simulink library "ddm"  (R2021b)
settings: Solver=VariableStepAuto  StartTime=0.0  StopTime=10.0  RelTol=1e-3
undefined symbols (not defined in the file or in its folder): ENUM_ADASACCSTA_ERROR, ENUM_ADASACCSTA_OFF, ENUM_ADASACCSTA_STANDBY, ENUM_ADASISASTA_OFF, ENUM_ALLOWMOV_ALLOWREADY, ENUM_APS, ENUM_BRKSTA_ERROR, ENUM_BRKSTA_OFF, ENUM_BRKSTA_ON, ENUM_CHGPREACTERRSTA_OBCPRE, ENUM_DCDCFAULTSTA_ANYFAULTLV1, ENUM_DCDCFAULTSTA_ANYFAULTLV2, ENUM_DRIVETRAIN_AWD, ENUM_DRIVETRAIN_FWD, ENUM_DRIVETRAIN_RWD, ENUM_DRSEATSTA_INVALID, ENUM_EDUDRTSTA_NORMAL, ENUM_EPBSTA_APPLIED, ENUM_EPBSTA_RELEASED, ENUM_HVBATTREADYPRE_READY, ENUM_MCUWARN_LV0, ENUM_MCUWARN_LV1, ENUM_MCUWARN_LV2, ENUM_MCUWARN_LV3, ENUM_MCUWARN_NOERROR, ENUM_OBCFAULTSTA_ANYFAULT, ENUM_PAS_R2F2, ENUM_PDFAULT_BATTPDFAIL, ENUM_PDFAULT_DCDCDISABLE, ENUM_PDFAULT_MCUDISABLE, ENUM_PDFAULT_MCUDISCHRG, ENUM_POWERSTA_OFF, ENUM_POWERSTA_ON, ENUM_POWERSTA_READY, ENUM_POWERSTA_STANDBY, ENUM_PRESSINDI_LOW, ENUM_PUFAULT_BATTUPFAIL, ENUM_PUFAULT_DCDCENABLEFAIL, ENUM_PUFAULT_PRECHRGCHKFAIL, ENUM_PUFAULT_SAFETYCHKFAIL, ENUM_PUSTATE_COMPLETED, ENUM_PWRSTASW_OFF, ENUM_PWRSTASW_OFFA, ENUM_PWRSTASW_OFFCHVCHRG, ENUM_PWRSTASW_OFFCLVCHRG, ENUM_PWRSTASW_ON, ENUM_PWRSTASW_ONHVCHRG, ENUM_PWRSTASW_READY, ENUM_PWRSTASW_STANDBY, ENUM_RANGESTA_12IN, ENUM_RANGESTA_12OUT, ENUM_SHIFTCOMMAND_D, ENUM_SHIFTCOMMAND_N, ENUM_SHIFTCOMMAND_P, ENUM_SHIFTCOMMAND_R, ENUM_ZONEMALFUNLV_1ST, ENUM_ZONEMALFUNLV_2ND, ENUM_ZONEMALFUNLV_3RD, ENUM_ZONEMALFUNLV_4TH, ENUM_ZONESPDCTRLMODE_ACC ... (+832)
libraries: hcu_lib x738, $bdroot x26, simulink x7
(part 18 of 25)

== system ddm/DDM/DDM/PMM/SW failure/Tailgate switch failure ==
  note: Fail Safe During Detection
  note: Fail Safe After Decision
  note: Release Condition After Decision
  note: Release Condition During Detection
  note: Diagnostics and Fault Handling
  note: Test Detection Criteria
  note: Test Pass Criteria
  task_time_s : Inport
  VPMM_PowerSta_enum : Inport  Port=2
  VPMM_PwrStaSW_enum : Inport  Port=3
  VINP_TailgaSW : Inport  Port=4
  DTC_clear_request : Inport  Port=5
  Add2 : Sum
  Add3 : Sum
  Add4 : Sum  AccumDataTypeStr=uint16
  Constant{1..2,12..13,31} (5 alike) : Constant  Value=ZERO_INT
  Constant14 : Constant  Value=KDDM_TailgaSW_s
  Constant28 : Constant  Value=ZERO_FLOAT
  Constant29 : Constant  Value=ONE_INT
  Constant3 : Constant  Value=ONE_INT
  Constant37 : Constant  Value=ENUM_PWRSTASW_OFF
  Constant39 : Constant  Value=KDDM_TailgaSWPassTO_s
  Constant4 : Constant  Value=KDDM_TailgaSW_s
  Constant{42,47,52,54} (4 alike) : Constant  Value=TRUE
  Constant45 : Constant  Value=ENUM_POWERSTA_OFF
  Constant49 : Constant  Value=KDDM_TailgaSW_s
  Constant5 : Constant  Value=KDDM_TailgaSWPassTO_s
  Constant50 : Constant  Value=ENUM_PWRSTASW_OFF
  Constant53 : Constant  Value=FALSE
  Constant55 : Constant  Value=FALSE
  Constant56 : Constant  Value=KDDM_TailgaSWPassSW_flg
  Constant57 : Constant  Value=KDDM_TailgaSWCFSSW_flg
  Constant58 : Constant  Value=KDDM_TailgaSWDFSSW_flg
  Constant59 : Constant  Value=KDDM_TailgaSWDetSW_flg
  Constant6 : Constant  Value=KDDM_TailgaSWDetTO_s
  Constant60 : Constant  Value=KDDM_TailgaSWDTC_cnt
  Constant7 : Constant  Value=KDDM_TailgaSWDetTO_s
  Constant8 : Constant  Value=KDDM_TailgaSWDTC_cnt
  Constant9 : Constant  Value=FALSE
  DTC_Couter1 : hcu_lib/Basic_Blocks/DTC_Couter
  DTC_Info : hcu_lib/Basic_Blocks/DTC_Info
  Data Type Conversion : DataTypeConversion  OutDataTypeStr=uint8
  Data Type Conversion{1..2,7..9} (5 alike) : DataTypeConversion
  Data Type Conversion3 : DataTypeConversion  OutDataTypeStr=uint16
  Data Type Conversion4 : DataTypeConversion  OutDataTypeStr=uint8
  Data Type Conversion5 : DataTypeConversion  OutDataTypeStr=uint32
  Data Type Conversion6 : DataTypeConversion  OutDataTypeStr=uint16
  Divide{,1,7,11,16,20} (6 alike) : Product  Inputs=*/
  Equal10 : RelationalOperator  Operator=~=  OutDataTypeStr=boolean  RndMeth=Simplest
  Equal13 : RelationalOperator  Operator=~=  OutDataTypeStr=boolean  RndMeth=Simplest
  Equal8 : RelationalOperator  Operator===  OutDataTypeStr=boolean  RndMeth=Simplest
  Equal9 : RelationalOperator  Operator=~=  OutDataTypeStr=boolean  RndMeth=Simplest
  Logical Operator1 : Logic  Operator=NOT  AllPortsSameDT=off  OutDataTypeStr=boolean
  Logical Operator{25,28..31} (5 alike) : Logic  AllPortsSameDT=off  OutDataTypeStr=boolean
  Logical Operator27 : Logic  Operator=OR  AllPortsSameDT=off  OutDataTypeStr=boolean
  Logical Operator32 : Logic  Operator=OR  AllPortsSameDT=off  OutDataTypeStr=boolean
  Logical Operator33 : Logic  Operator=OR  AllPortsSameDT=off  OutDataTypeStr=boolean
  Relational Operator : RelationalOperator  Operator=>  OutDataTypeStr=boolean  RndMeth=Simplest
  Relational Operator1 : RelationalOperator  Operator=<=  OutDataTypeStr=boolean  RndMeth=Simplest
  Relational Operator12 : RelationalOperator  OutDataTypeStr=boolean  RndMeth=Simplest
  Relational Operator13 : RelationalOperator  Operator=<  OutDataTypeStr=boolean  RndMeth=Simplest
  Relational Operator2 : RelationalOperator  Operator=>  OutDataTypeStr=boolean  RndMeth=Simplest
  Relational Operator8 : RelationalOperator  Operator=<  OutDataTypeStr=boolean  RndMeth=Simplest
  Relational Operator9 : RelationalOperator  Operator=<=  OutDataTypeStr=boolean  RndMeth=Simplest
  Relay1 : Relay  OnSwitchValue=ONE_INT  OffSwitchValue=ZERO_INT
  SR_Latch2 : hcu_lib/Basic_Blocks/SR_Latch
  SR_Latch5 : hcu_lib/Basic_Blocks/SR_Latch
  Switch{1..3,6,8..9,13} (7 alike) : Switch  Criteria=u2 > Threshold
  Switch{4,7,11..12,15..16} (6 alike) : Switch  Criteria=u2 ~= 0
  Test Detection Criteria1 : hcu_lib/Basic_Blocks/Test Detection Criteria
  Unit Delay{1..3,5..6} (5 alike) : UnitDelay  SampleTime=-1  HasFrameUpgradeWarning=on
  VDDM_TailgaSWDTC_raw32 : Outport
  VCUTailgaSWSta : Outport  Port=2
  wires:
  DTC_clear_request/1 -> [DTC_clear_request]
  VINP_TailgaSW/1 -> [VINP_TailgaSWGPIO_flg]
  task_time_s/1 -> [task_time_s]
  [VDDM_TailgaSWCFS_flg] -> Switch11/2
  Constant42/1 -> Switch11/1
  Switch11/1 -> [VCUTailgaSWSta]
  Logical Operator27/1 -> Switch15/2
  Constant52/1 -> Switch16/1
  Equal8/1 -> Logical Operator27/1
  [VDDM_TailgaSWPass_flg] -> Switch16/2
  Constant53/1 -> Switch16/3
  Constant45/1 -> Equal8/2
  Constant55/1 -> Switch15/3
  Switch15/1 -> [VDDM_TailgaSWCFSRls_flg]
  Switch16/1 -> [VDDM_TailgaSWDFSRls_flg]
  [DTC_clear_request] -> Logical Operator27/2
  Constant54/1 -> Switch15/1
  [VPMM_PowerSta_enum] -> Equal8/1
  Relay1/1 -> SR_Latch2/1
  [VDDM_TailgaSWDet_flg] -> Logical Operator31/1
  Logical Operator29/1 -> DTC_Couter1/2
  [VDDM_TailgaSWCFSRls_flg] -> SR_Latch5/2
  SR_Latch2/1 -> Logical Operator28/2
  SR_Latch5/1 -> Logical Operator30/1
  [VDDM_TailgaSWDFSRls_flg] -> Logical Operator32/1
  Logical Operator32/1 -> SR_Latch2/2
  DTC_Couter1/2 -> Data Type Conversion4/1
  Logical Operator33/1 -> Logical Operator29/1
  Data Type Conversion4/1 -> [VDDM_TailgaSWDTC_cnt]  "VDDM_TailgaSWDTC_cnt"
  [VDDM_TailgaSWDTC_cnt] -> Relay1/1
  Logical Operator31/1 -> DTC_Couter1/1
  [VDDM_TailgaSWCFS_flg] -> Logical Operator32/2
  Constant57/1 -> Logical Operator30/2
  DTC_Couter1/1 -> SR_Latch5/1
  Constant59/1 -> Logical Operator31/2
  [VDDM_TailgaSWCFSRls_flg] -> Logical Operator33/2
  Logical Operator28/1 -> [VDDM_TailgaSWDFS_flg]
  [VDDM_TailgaSWPass_flg] -> Logical Operator33/1
  Logical Operator30/1 -> [VDDM_TailgaSWCFS_flg]
  Constant56/1 -> Logical Operator29/2
  Constant60/1 -> DTC_Couter1/3
  Constant58/1 -> Logical Operator28/1
  [VCUTailgaSWSta] -> VCUTailgaSWSta/1
  Divide1/1 -> Relational Operator1/2
  Data Type Conversion5/1 -> [VDDM_TailgaSWHiLoCount_enum]
  Relational Operator1/1 -> [VDDM_TailgaSWFailcntEN_flg]
  Divide20/1 -> Data Type Conversion9/1
  Add2/1 -> Switch6/3
  [VINP_TailgaSWGPIO_flg] -> Relational Operator/1
  Relational Operator2/1 -> Switch1/2
  Constant31/1 -> Switch6/1
  Unit Delay3/1 -> Equal10/1
  Equal10/1 -> [VDDM_TailgaSWChange_flg]
  Constant1/1 -> Switch7/3
  Constant29/1 -> Add2/2
  Switch6/1 -> Unit Delay1/1
  Unit Delay1/1 -> Data Type Conversion5/1
  Constant12/1 -> Switch1/1
  Constant37/1 -> Equal13/2
  Switch2/1 -> Data Type Conversion2/1
  Add3/1 -> Data Type Conversion8/1
  Constant4/1 -> Divide/1
  Switch9/1 -> Switch8/1
  Equal13/1 -> Switch7/2
  [VDDM_TailgaSWfail_cnt] -> Switch1/3
  [VPMM_PwrStaSW_enum] -> Equal13/1
  Switch7/1 -> Unit Delay5/1
  [VDDM_TailgaSWHiLoCount_enum] -> Relational Operator2/1
  [VDDM_TailgaSWFailcntEN_flg] -> Switch9/2
  Switch1/1 -> Switch8/3
  Test Detection Criteria1/1 -> [VDDM_TailgaSWDet_flg]  "VDDM_TailgaSWDet_flg"
  Constant7/1 -> Test Detection Criteria1/4
  [VDDM_TailgaSWHiLoCount_enum] -> Add3/1
  [VDDM_TailgaSWChange_flg] -> Switch6/2
  [VDDM_TailgaSWfail_cnt] -> Switch2/1, Relational Operator8/1
  Constant13/1 -> Switch9/3
  Constant14/1 -> Divide1/1
  Relational Operator/1 -> Unit Delay3/1, Equal10/2
  Constant28/1 -> Relational Operator/2
  Constant6/1 -> Divide20/1
  [VDDM_TailgaSWChange_flg] -> Switch8/2
  Switch8/1 -> Switch7/1
  Divide/1 -> Relational Operator2/2
  Unit Delay2/1 -> Relational Operator9/1
  Switch12/1 -> Unit Delay6/1
  Constant3/1 -> Add4/1
  Relational Operator9/1 -> Logical Operator25/2
  Data Type Conversion6/1 -> Relational Operator12/1, [VDDM_TailgaSWPass_cnt]
  [VDDM_TailgaSWChange_flg] -> Logical Operator25/1
  Switch3/1 -> Data Type Conversion3/1
  Constant2/1 -> Switch13/3
  [VDDM_TailgaSWPass_cnt] -> Switch3/1, Relational Operator13/1
  Divide11/1 -> Relational Operator12/2
  Logical Operator1/1 -> Switch13/2
  Logical Operator25/1 -> Logical Operator1/1
  Data Type Conversion/1 -> Switch12/3
  Constant5/1 -> Divide11/1
  Data Type Conversion3/1 -> Add4/2
  Add4/1 -> Switch13/1
  Equal9/1 -> Switch12/2
  Relational Operator12/1 -> [VDDM_TailgaSWPass_flg]
  Switch13/1 -> Switch12/1
  Divide7/1 -> Relational Operator9/2
  [VPMM_PwrStaSW_enum] -> Equal9/1
  Constant50/1 -> Equal9/2
  Unit Delay6/1 -> Data Type Conversion6/1
  Constant47/1 -> Data Type Conversion/1
  Constant49/1 -> Divide7/1
  Constant39/1 -> Divide16/1
  [VDDM_TailgaSWHiLoCount_enum] -> Unit Delay2/1
  VPMM_PwrStaSW_enum/1 -> [VPMM_PwrStaSW_enum]
  VPMM_PowerSta_enum/1 -> [VPMM_PowerSta_enum]
  [VINP_TailgaSWGPIO_flg] -> Switch11/3
  Data Type Conversion9/1 -> Switch2/3, Relational Operator8/2
  Relational Operator8/1 -> Switch2/2
  Data Type Conversion2/1 -> Add3/2
  [VDDM_TailgaSWHiLoCount_enum] -> Relational Operator1/1
  [VDDM_TailgaSWHiLoCount_enum] -> Add2/1
  Data Type Conversion7/1 -> [VDDM_TailgaSWfail_cnt]
  Relational Operator13/1 -> Switch3/2
  Divide16/1 -> Data Type Conversion1/1
  Data Type Conversion1/1 -> Switch3/3, Relational Operator13/2
  Data Type Conversion8/1 -> Switch9/1
  DTC_Info/1 -> VDDM_TailgaSWDTC_raw32/1  "VDDM_TailgaSWDTC_raw32"
  [VDDM_TailgaSWPass_flg] -> DTC_Info/2
  [VDDM_TailgaSWCFS_flg] -> DTC_Info/3
  [VDDM_TailgaSWDet_flg] -> DTC_Info/1
  [task_time_s] -> Divide1/2
  [task_time_s] -> Divide20/2
  [task_time_s] -> Divide/2
  [task_time_s] -> Test Detection Criteria1/2
  [task_time_s] -> Divide16/2
  [task_time_s] -> Divide7/2
  [task_time_s] -> Divide11/2
  Constant8/1 -> Test Detection Criteria1/3
  [DTC_clear_request] -> DTC_Info/4
  [DTC_clear_request] -> Switch4/2
  Switch4/1 -> Test Detection Criteria1/1
  Unit Delay5/1 -> Data Type Conversion7/1, Switch4/3
  Constant9/1 -> Switch4/1

== system ddm/DDM/DDM/PMM/System conditions of ON to READY not satisfied/SR_Latch1 ==
  set : Inport
  reset : Inport  Port=2
  Logical Operator : Logic  AllPortsSameDT=off  OutDataTypeStr=boolean
  Logical Operator1 : Logic  Operator=NOT  AllPortsSameDT=off  OutDataTypeStr=boolean
  Switch1 : Switch  Criteria=u2 ~= 0  Threshold=0.5
      settings: AttributesFormatString=<Criteria=%<Criteria>>
  Switch2 : Switch  Criteria=u2 ~= 0  Threshold=0.5
      settings: AttributesFormatString=<Criteria=%<Criteria>>
  Unit Delay : UnitDelay  SampleTime=-1  HasFrameUpgradeWarning=on
  latched : Outport
  wires:
  Logical Operator1/1 -> Switch2/1, Logical Operator/2
  Logical Operator/1 -> Switch1/2
  Switch2/1 -> Switch1/3
  Unit Delay/1 -> Switch2/3
  reset/1 -> Logical Operator1/1, Switch2/2
  set/1 -> Logical Operator/1, Switch1/1
  Switch1/1 -> latched/1, Unit Delay/1

== system ddm/DDM/DDM/PMM/power up and power down/BMS HV relay closed fail ==
  note: Release Condition After Failure Decision
  note: Test Detection Criteria
  note: Test Pass Criteria
  note: Release Condition During Failure Detection
  note: Diagnostics and Fault Handling
  note: Fail Safe Operation During Failure Detection
  note: Fail Safe Operation After Failure Decision
  task_time_s : Inport
  VPMM_PowerSta_enum : Inport  Port=2
  VPMM_PwrStaSW_enum : Inport  Port=3
  VINP_HVBContactorSta_flg : Inport  Port=4
  VPMM_PowerUpFault_enum : Inport  Port=5
  DTC_clear_request : Inport  Port=6
  VPMM_PowerUpState_enum : Inport  Port=7
  Constant : Constant  Value=ENUM_PUFAULT_BATTUPFAIL
  Constant1 : Constant  Value=ENUM_PUSTATE_COMPLETED
  Constant10 : Constant  Value=KDDM_HVRlyCloDTC_cnt
  Constant11 : Constant  Value=KDDM_HVRlyCloPassSW_flg
  Constant15 : Constant  Value=KDDM_HVRlyCloCFSSW_flg
  Constant16 : Constant  Value=TRUE
  Constant19 : Constant  Value=ENUM_POWERSTA_OFF
  Constant{2,21,25,27} (4 alike) : Constant  Value=FALSE
  Constant20 : Constant  Value=KDDM_HVRlyCloDFSSW_flg
  Constant23 : Constant  Value=TRUE
  Constant24 : Constant  Value=TRUE
  Constant26 : Constant  Value=ENUM_PWRSTASW_OFF
  Constant38 : Constant  Commented=on  Value=KDDM_HVRlyCloDetTO_s
  Constant40 : Constant  Commented=on  Value=KDDM_HVRlyCloDTC_cnt
  Constant43 : Constant  Value=KDDM_HVRlyCloPassTO_s
  Constant44 : Constant  Value=KDDM_HVRlyCloDetSW_flg
  Constant8 : Constant  Value=KDDM_HVRlyCloPassTO_s
  DTC_Couter : hcu_lib/Basic_Blocks/DTC_Couter
  DTC_Info : hcu_lib/Basic_Blocks/DTC_Info
  Data Type Conversion1 : DataTypeConversion  OutDataTypeStr=uint8
  Equal : RelationalOperator  Operator=~=  OutDataTypeStr=boolean  RndMeth=Simplest
  Equal1 : RelationalOperator  Operator===  OutDataTypeStr=boolean  RndMeth=Simplest
  Equal2 : RelationalOperator  Operator===  OutDataTypeStr=boolean  RndMeth=Simplest
  Equal5 : RelationalOperator  OutDataTypeStr=boolean  RndMeth=Simplest
  Equal6 : RelationalOperator  Operator===  OutDataTypeStr=boolean  RndMeth=Simplest
  From48 : From  Commented=on  GotoTag=task_time_s
  Goto24 : Goto  Commented=on  GotoTag=VDDM_EDriveSysErrVCUErr_flg
  Logical Operator{5,12,15,18..19} (5 alike) : Logic  AllPortsSameDT=off  OutDataTypeStr=boolean
  Logical Operator3 : Logic  Operator=OR  AllPortsSameDT=off  OutDataTypeStr=boolean
  Logical Operator4 : Logic  Operator=NOT  AllPortsSameDT=off  OutDataTypeStr=boolean
  Logical Operator6 : Logic  Operator=NOT  AllPortsSameDT=off  OutDataTypeStr=boolean
  Logical Operator8 : Logic  Operator=OR  AllPortsSameDT=off  OutDataTypeStr=boolean
  Relay : Relay  OnSwitchValue=ONE_INT  OffSwitchValue=ZERO_INT
  SR_Latch1 : Subsystem  mask(SR_Latch){}
      mask help: SR latch function.
  SR_Latch3 : hcu_lib/Basic_Blocks/SR_Latch
  SR_Latch4 : hcu_lib/Basic_Blocks/SR_Latch
  Switch{,2,4..5} (4 alike) : Switch  Criteria=u2 ~= 0
  Test Detection Criteria : hcu_lib/Basic_Blocks/Test Detection Criteria  Commented=on
  Timer1 : hcu_lib/Basic_Blocks/Timer
  VDDM_HVRlyCloDTC_raw32 : Outport
  wires:
  task_time_s/1 -> [task_time_s]
  VPMM_PwrStaSW_enum/1 -> [VPMM_PwrStaSW_enum]
  VPMM_PowerSta_enum/1 -> [VPMM_PowerSta_enum]
  Logical Operator18/1 -> [VDDM_HVRlyCloCFS_flg]
  Constant21/1 -> Switch/3
  Equal5/1 -> SR_Latch1/1(set)
  Switch4/1 -> [VDDM_HVRlyCloCFSRls_flg]
  Data Type Conversion1/1 -> [VDDM_HVRlyCloDTC_cnt]  "VDDM_HVRlyCloDTC_cnt"
  Constant8/1 -> Equal5/2
  Constant20/1 -> Logical Operator12/1
  Logical Operator12/1 -> [VDDM_HVRlyCloDFS_flg]
  Constant15/1 -> Logical Operator18/2
  [task_time_s] -> Timer1/3
  DTC_Couter/1 -> SR_Latch4/1
  [VDDM_HVRlyCloCFSRls_flg] -> Logical Operator3/2
  Logical Operator19/1 -> DTC_Couter/1
  [VPMM_PowerSta_enum] -> Equal6/1
  [VDDM_HVRlyCloPass_flg] -> Logical Operator3/1
  Constant23/1 -> Switch2/3
  Constant16/1 -> Switch/1
  Constant26/1 -> Equal/2
  SR_Latch3/1 -> Logical Operator12/2
  From48/1 -> Test Detection Criteria/2
  Switch/1 -> Goto24/1
  Switch5/1 -> [VDDM_HVRlyCloDet_flg]  "VDDM_HVRlyCloDet_flg"
  [VDDM_HVRlyCloDet_flg] -> Logical Operator19/1
  Logical Operator3/1 -> Logical Operator15/1
  Constant24/1 -> Switch4/1
  SR_Latch4/1 -> Logical Operator18/1
  Logical Operator15/1 -> DTC_Couter/2
  Constant10/1 -> DTC_Couter/3
  Constant40/1 -> Test Detection Criteria/3
  Constant25/1 -> Switch4/3
  [VPMM_PwrStaSW_enum] -> Equal/1
  Relay/1 -> SR_Latch3/1
  [VDDM_HVRlyCloCFS_flg] -> Switch/2
  [DTC_clear_request] -> Logical Operator8/2
  Constant11/1 -> Logical Operator15/2
  [VDDM_HVRlyCloDTC_cnt] -> Relay/1
  Equal2/1 -> Switch2/2
  Equal/1 -> Switch5/2
  Logical Operator8/1 -> Switch4/2
  Logical Operator6/1 -> Timer1/1
  SR_Latch1/1(latched) -> [VDDM_HVRlyCloPass_flg]
  Equal6/1 -> Logical Operator8/1
  Constant27/1 -> Switch5/3
  Constant43/1 -> Timer1/4
  DTC_Couter/2 -> Data Type Conversion1/1
  Constant44/1 -> Logical Operator19/2
  Constant19/1 -> Equal6/2
  [VDDM_HVRlyCloChk_flg] -> Switch5/1
  Timer1/1 -> Equal5/1
  Switch2/1 -> SR_Latch1/2(reset), Timer1/2, Logical Operator6/1
  [VDDM_HVRlyCloCFSRls_flg] -> SR_Latch4/2
  DTC_clear_request/1 -> [DTC_clear_request]
  Constant/1 -> Equal1/2
  Equal1/1 -> Logical Operator5/2
  Logical Operator4/1 -> Logical Operator5/1
  VINP_HVBContactorSta_flg/1 -> Logical Operator4/1
  VPMM_PowerUpFault_enum/1 -> Equal1/1
  Logical Operator5/1 -> [VDDM_HVRlyCloChk_flg]
  DTC_Info/1 -> VDDM_HVRlyCloDTC_raw32/1  "VDDM_HVRlyCloDTC_raw32"
  [VDDM_HVRlyCloPass_flg] -> DTC_Info/2
  [VDDM_HVRlyCloCFS_flg] -> DTC_Info/3
  [VDDM_HVRlyCloCFS_flg] -> SR_Latch3/2
  [VDDM_HVRlyCloDet_flg] -> DTC_Info/1
  Constant38/1 -> Test Detection Criteria/4
  [DTC_clear_request] -> DTC_Info/4
  VPMM_PowerUpState_enum/1 -> [VPMM_PowerUpState_enum]
  Constant2/1 -> Switch2/1
  Constant1/1 -> Equal2/2
  [VPMM_PowerUpState_enum] -> Equal2/1

== system ddm/DDM/DDM/PMM/power up and power down/BMS HV relay opened fail ==
  note: Test Pass Criteria
  note: Diagnostics and Fault Handling
  note: Test Detection Criteria
  note: Fail Safe Operation After Failure Decision
  note: Release Condition During Failure Detection
  note: Fail Safe Operation During Failure Detection
  note: Release Condition After Failure Decision
  task_time_s : Inport
  VPMM_PowerSta_enum : Inport  Port=2
  VPMM_PwrStaSW_enum : Inport  Port=3
  VPMM_PowerDownFault_enum : Inport  Port=4
  DTC_clear_request : Inport  Port=5
  Constant : Constant  Value=ENUM_PDFAULT_BATTPDFAIL
  Constant1 : Constant  Value=ENUM_PWRSTASW_OFF
  Constant10 : Constant  Value=KDDM_HVRlyOpDTC_cnt
  Constant11 : Constant  Value=KDDM_HVRlyOpPassSW_flg
  Constant15 : Constant  Value=KDDM_HVRlyOpCFSSW_flg
  Constant16 : Constant  Value=TRUE
  Constant17 : Constant  Value=KDDM_HVRlyOpPassTO_s
  Constant19 : Constant  Value=ENUM_POWERSTA_OFF
  Constant20 : Constant  Value=KDDM_HVRlyOpDFSSW_flg
  Constant21 : Constant  Value=FALSE
  Constant22 : Constant  Value=ENUM_PWRSTASW_OFF
  Constant23 : Constant  Value=TRUE
  Constant24 : Constant  Value=TRUE
  Constant25 : Constant  Value=FALSE
  Constant27 : Constant  Value=FALSE
  Constant38 : Constant  Commented=on  Value=KDDM_HVRlyOpDetTO_s
  Constant40 : Constant  Commented=on  Value=KDDM_HVRlyOpDTC_cnt
  Constant43 : Constant  Value=KDDM_HVRlyOpPassTO_s
  Constant44 : Constant  Value=KDDM_HVRlyOpDetSW_flg
  DTC_Couter : hcu_lib/Basic_Blocks/DTC_Couter
  DTC_Info : hcu_lib/Basic_Blocks/DTC_Info
  Data Type Conversion1 : DataTypeConversion  OutDataTypeStr=uint8
  Equal1 : RelationalOperator  Operator===  OutDataTypeStr=boolean  RndMeth=Simplest
  Equal2 : RelationalOperator  Operator=~=  OutDataTypeStr=boolean  RndMeth=Simplest
  Equal4 : RelationalOperator  Operator=~=  OutDataTypeStr=boolean  RndMeth=Simplest
  Equal6 : RelationalOperator  OutDataTypeStr=boolean  RndMeth=Simplest
  Equal7 : RelationalOperator  Operator===  OutDataTypeStr=boolean  RndMeth=Simplest
  From48 : From  Commented=on  GotoTag=task_time_s
  Logical Operator{12,15,18..19} (4 alike) : Logic  AllPortsSameDT=off  OutDataTypeStr=boolean
  Logical Operator3 : Logic  Operator=OR  AllPortsSameDT=off  OutDataTypeStr=boolean
  Logical Operator6 : Logic  Operator=NOT  AllPortsSameDT=off  OutDataTypeStr=boolean
  Logical Operator8 : Logic  Operator=OR  AllPortsSameDT=off  OutDataTypeStr=boolean
  Relay : Relay  OnSwitchValue=ONE_INT  OffSwitchValue=ZERO_INT
  SR_Latch1 : Subsystem  mask(SR_Latch){}
      mask help: SR latch function.
  SR_Latch3 : hcu_lib/Basic_Blocks/SR_Latch
  SR_Latch4 : hcu_lib/Basic_Blocks/SR_Latch
  Switch{,1,4..5} (4 alike) : Switch  Criteria=u2 ~= 0
  Test Detection Criteria : hcu_lib/Basic_Blocks/Test Detection Criteria  Commented=on
  Timer1 : hcu_lib/Basic_Blocks/Timer
  VDDM_HVRlyOpDTC_raw32 : Outport
  VDDM_HVRlyOpFail_flg : Outport  Port=2
  wires:
  task_time_s/1 -> [task_time_s]
  VPMM_PwrStaSW_enum/1 -> [VPMM_PwrStaSW_enum]
  VPMM_PowerSta_enum/1 -> [VPMM_PowerSta_enum]
  Equal4/1 -> Switch5/2
  SR_Latch1/1(latched) -> [VDDM_HVRlyOpPass_flg]
  Constant44/1 -> Logical Operator19/2
  [VDDM_HVRlyOpDTC_cnt] -> Relay/1
  Equal2/1 -> Switch1/2
  [VDDM_HVRlyOpCFSRls_flg] -> SR_Latch4/2
  DTC_Couter/2 -> Data Type Conversion1/1
  Constant20/1 -> Logical Operator12/1
  SR_Latch4/1 -> Logical Operator18/1
  Constant23/1 -> Switch1/3
  Constant11/1 -> Logical Operator15/2
  Constant17/1 -> Equal6/2
  Logical Operator15/1 -> DTC_Couter/2
  DTC_Couter/1 -> SR_Latch4/1
  Constant27/1 -> Switch5/3
  [VPMM_PwrStaSW_enum] -> Equal4/1
  [VPMM_PowerSta_enum] -> Equal7/1
  Switch4/1 -> [VDDM_HVRlyOpCFSRls_flg]
  [VDDM_HVRlyOpChk_flg] -> Switch1/1
  [VDDM_HVRlyOpCFS_flg] -> Switch/2
  Constant19/1 -> Equal7/2
  Constant21/1 -> Switch/3
  [VDDM_HVRlyOpDet_flg] -> Logical Operator19/1
  Logical Operator3/1 -> Logical Operator15/1
  [VDDM_HVRlyOpChk_flg] -> Switch5/1
  [task_time_s] -> Timer1/3
  Constant43/1 -> Timer1/4
  Constant22/1 -> Equal4/2
  Constant25/1 -> Switch4/3
  Relay/1 -> SR_Latch3/1
  Timer1/1 -> Equal6/1
  Constant10/1 -> DTC_Couter/3
  Switch1/1 -> Logical Operator6/1, SR_Latch1/2(reset), Timer1/2
  Equal6/1 -> SR_Latch1/1(set)
  Logical Operator18/1 -> [VDDM_HVRlyOpCFS_flg]
  Data Type Conversion1/1 -> [VDDM_HVRlyOpDTC_cnt]  "VDDM_HVRlyOpDTC_cnt"
  Constant24/1 -> Switch4/1
  From48/1 -> Test Detection Criteria/2
  Switch/1 -> [VDDM_HVRlyOpFail_flg]  "VDDM_HVRlyOpFail_flg"
  SR_Latch3/1 -> Logical Operator12/2
  [VDDM_HVRlyOpCFSRls_flg] -> Logical Operator3/2
  Logical Operator6/1 -> Timer1/1
  [VDDM_HVRlyOpPass_flg] -> Logical Operator3/1
  Logical Operator8/1 -> Switch4/2
  Constant40/1 -> Test Detection Criteria/3
  Switch5/1 -> [VDDM_HVRlyOpDet_flg]  "VDDM_HVRlyOpDet_flg"
  Constant1/1 -> Equal2/2
  Logical Operator12/1 -> [VDDM_HVRlyOpDFS_flg]
  Equal7/1 -> Logical Operator8/1
  [VPMM_PwrStaSW_enum] -> Equal2/1
  Constant16/1 -> Switch/1
  Constant15/1 -> Logical Operator18/2
  [DTC_clear_request] -> Logical Operator8/2
  Logical Operator19/1 -> DTC_Couter/1
  DTC_clear_request/1 -> [DTC_clear_request]
  VPMM_PowerDownFault_enum/1 -> Equal1/1
  Constant/1 -> Equal1/2
  Equal1/1 -> [VDDM_HVRlyOpChk_flg]
  [VDDM_HVRlyOpFail_flg] -> VDDM_HVRlyOpFail_flg/1
  DTC_Info/1 -> VDDM_HVRlyOpDTC_raw32/1  "VDDM_HVRlyOpDTC_raw32"
  [VDDM_HVRlyOpPass_flg] -> DTC_Info/2
  [VDDM_HVRlyOpCFS_flg] -> DTC_Info/3
  [VDDM_HVRlyOpCFS_flg] -> SR_Latch3/2
  [VDDM_HVRlyOpDet_flg] -> DTC_Info/1
  Constant38/1 -> Test Detection Criteria/4
  [DTC_clear_request] -> DTC_Info/4

== system ddm/DDM/DDM/PMM/power up and power down/BMS ready fail ==
  note: Fail Safe Operation After Failure Decision
  note: Fail Safe Operation During Failure Detection
  note: Diagnostics and Fault Handling
  note: Release Condition During Failure Detection
  note: Test Pass Criteria
  note: Test Detection Criteria
  note: Release Condition After Failure Decision
  task_time_s : Inport
  VPMM_PowerSta_enum : Inport  Port=2
  VPMM_PwrStaSW_enum : Inport  Port=3
  VINP_BMSREADY_flg : Inport  Port=4
  VPMM_PowerUpFault_enum : Inport  Port=5
  DTC_clear_request : Inport  Port=6
  VPMM_PowerUpState_enum : Inport  Port=7
  Constant : Constant  Value=ENUM_PUFAULT_BATTUPFAIL
  Constant1 : Constant  Value=ENUM_PWRSTASW_OFF
  Constant10 : Constant  Value=KDDM_BMSRdyDTC_cnt
  Constant11 : Constant  Value=KDDM_BMSRdyPassSW_flg
  Constant15 : Constant  Value=KDDM_BMSRdyCFSSW_flg
  Constant16 : Constant  Value=TRUE
  Constant19 : Constant  Value=ENUM_POWERSTA_OFF
  Constant2 : Constant  Value=ENUM_PUSTATE_COMPLETED
  Constant20 : Constant  Value=KDDM_BMSRdyDFSSW_flg
  Constant{3,21,25,27} (4 alike) : Constant  Value=FALSE
  Constant23 : Constant  Value=TRUE
  Constant24 : Constant  Value=TRUE
  Constant38 : Constant  Commented=on  Value=KDDM_BMSRdyDetTO_s
  Constant40 : Constant  Commented=on  Value=KDDM_BMSRdyDTC_cnt
  Constant43 : Constant  Value=KDDM_BMSRdyPassTO_s
  Constant44 : Constant  Value=KDDM_BMSRdyDetSW_flg
  Constant8 : Constant  Value=KDDM_BMSRdyPassTO_s
  DTC_Couter : hcu_lib/Basic_Blocks/DTC_Couter
  DTC_Info : hcu_lib/Basic_Blocks/DTC_Info
  Data Type Conversion1 : DataTypeConversion  OutDataTypeStr=uint8
  Equal : RelationalOperator  Operator=~=  OutDataTypeStr=boolean  RndMeth=Simplest
  Equal1 : RelationalOperator  Operator===  OutDataTypeStr=boolean  RndMeth=Simplest
  Equal2 : RelationalOperator  Operator===  OutDataTypeStr=boolean  RndMeth=Simplest
  Equal5 : RelationalOperator  OutDataTypeStr=boolean  RndMeth=Simplest
  Equal6 : RelationalOperator  Operator===  OutDataTypeStr=boolean  RndMeth=Simplest
  From48 : From  Commented=on  GotoTag=task_time_s
  Goto24 : Goto  Commented=on  GotoTag=VDDM_EDriveSysErrVCUErr_flg
  Logical Operator{5,12,15,18..19} (5 alike) : Logic  AllPortsSameDT=off  OutDataTypeStr=boolean
  Logical Operator3 : Logic  Operator=OR  AllPortsSameDT=off  OutDataTypeStr=boolean
  Logical Operator4 : Logic  Operator=NOT  AllPortsSameDT=off  OutDataTypeStr=boolean
  Logical Operator6 : Logic  Operator=NOT  AllPortsSameDT=off  OutDataTypeStr=boolean
  Logical Operator8 : Logic  Operator=OR  AllPortsSameDT=off  OutDataTypeStr=boolean
  Relay : Relay  OnSwitchValue=ONE_INT  OffSwitchValue=ZERO_INT
  SR_Latch1 : Subsystem  mask(SR_Latch){}
      mask help: SR latch function.
  SR_Latch3 : hcu_lib/Basic_Blocks/SR_Latch
  SR_Latch4 : hcu_lib/Basic_Blocks/SR_Latch
  Switch{,2,4..5} (4 alike) : Switch  Criteria=u2 ~= 0
  Test Detection Criteria : hcu_lib/Basic_Blocks/Test Detection Criteria  Commented=on
  Timer1 : hcu_lib/Basic_Blocks/Timer
  VDDM_BMSRdyDTC_raw32 : Outport
  wires:
  Logical Operator5/1 -> [VDDM_BMSRdyChk_flg]
  VPMM_PowerUpFault_enum/1 -> Equal1/1
  VINP_BMSREADY_flg/1 -> Logical Operator4/1
  Logical Operator4/1 -> Logical Operator5/1
  Equal1/1 -> Logical Operator5/2
  Constant/1 -> Equal1/2
  DTC_clear_request/1 -> [DTC_clear_request]
  [VDDM_BMSRdyCFSRls_flg] -> SR_Latch4/2
  Switch2/1 -> Logical Operator6/1, Timer1/2, SR_Latch1/2(reset)
  Timer1/1 -> Equal5/1
  [VDDM_BMSRdyChk_flg] -> Switch5/1
  Constant19/1 -> Equal6/2
  Constant44/1 -> Logical Operator19/2
  DTC_Couter/2 -> Data Type Conversion1/1
  Constant43/1 -> Timer1/4
  Constant27/1 -> Switch5/3
  Equal6/1 -> Logical Operator8/1
  SR_Latch1/1(latched) -> [VDDM_BMSRdyPass_flg]
  Logical Operator6/1 -> Timer1/1
  Logical Operator8/1 -> Switch4/2
  Equal/1 -> Switch5/2
  Equal2/1 -> Switch2/2
  [VDDM_BMSRdyDTC_cnt] -> Relay/1
  Constant11/1 -> Logical Operator15/2
  [DTC_clear_request] -> Logical Operator8/2
  [VDDM_BMSRdyCFS_flg] -> Switch/2
  Relay/1 -> SR_Latch3/1
  [VPMM_PwrStaSW_enum] -> Equal/1
  Constant25/1 -> Switch4/3
  Constant40/1 -> Test Detection Criteria/3
  Constant10/1 -> DTC_Couter/3
  Logical Operator15/1 -> DTC_Couter/2
  SR_Latch4/1 -> Logical Operator18/1
  Constant24/1 -> Switch4/1
  Logical Operator3/1 -> Logical Operator15/1
  [VDDM_BMSRdyDet_flg] -> Logical Operator19/1
  Switch5/1 -> [VDDM_BMSRdyDet_flg]  "VDDM_BMSRdyDet_flg"
  Switch/1 -> Goto24/1
  From48/1 -> Test Detection Criteria/2
  SR_Latch3/1 -> Logical Operator12/2
  Constant1/1 -> Equal/2
  Constant16/1 -> Switch/1
  Constant23/1 -> Switch2/3
  [VDDM_BMSRdyPass_flg] -> Logical Operator3/1
  [VPMM_PowerSta_enum] -> Equal6/1
  Logical Operator19/1 -> DTC_Couter/1
  [VDDM_BMSRdyCFSRls_flg] -> Logical Operator3/2
  DTC_Couter/1 -> SR_Latch4/1
  [task_time_s] -> Timer1/3
  Constant15/1 -> Logical Operator18/2
  Logical Operator12/1 -> [VDDM_BMSRdyDFS_flg]
  Constant20/1 -> Logical Operator12/1
  Constant8/1 -> Equal5/2
  Data Type Conversion1/1 -> [VDDM_BMSRdyDTC_cnt]  "VDDM_BMSRdyDTC_cnt"
  Switch4/1 -> [VDDM_BMSRdyCFSRls_flg]
  Equal5/1 -> SR_Latch1/1(set)
  Constant21/1 -> Switch/3
  Logical Operator18/1 -> [VDDM_BMSRdyCFS_flg]
  VPMM_PowerSta_enum/1 -> [VPMM_PowerSta_enum]
  VPMM_PwrStaSW_enum/1 -> [VPMM_PwrStaSW_enum]
  task_time_s/1 -> [task_time_s]
  DTC_Info/1 -> VDDM_BMSRdyDTC_raw32/1  "VDDM_BMSRdyDTC_raw32"
  [VDDM_BMSRdyCFS_flg] -> DTC_Info/3
  [VDDM_BMSRdyCFS_flg] -> SR_Latch3/2
  [VDDM_BMSRdyDet_flg] -> DTC_Info/1
  [VDDM_BMSRdyPass_flg] -> DTC_Info/2
  Constant38/1 -> Test Detection Criteria/4
  [DTC_clear_request] -> DTC_Info/4
  VPMM_PowerUpState_enum/1 -> [VPMM_PowerUpState_enum]
  Constant3/1 -> Switch2/1
  Constant2/1 -> Equal2/2
  [VPMM_PowerUpState_enum] -> Equal2/1

== system ddm/DDM/DDM/PMM/power up and power down/DCDC disable fail ==
  note: Fail Safe Operation After Failure Decision
  note: Fail Safe Operation During Failure Detection
  note: Diagnostics and Fault Handling
  note: Release Condition After Failure Decision
  note: Release Condition During Failure Detection
  note: Test Detection Criteria
  note: Test Pass Criteria
  task_time_s : Inport
  VPMM_PowerSta_enum : Inport  Port=2
  VPMM_PwrStaSW_enum : Inport  Port=3
  VPMM_PowerDownFault_enum : Inport  Port=4
  DTC_clear_request : Inport  Port=5
  Constant : Constant  Value=ENUM_PDFAULT_DCDCDISABLE
  Constant1 : Constant  Value=ENUM_PWRSTASW_OFF
  Constant10 : Constant  Value=KDDM_DCDCDisDTC_cnt
  Constant11 : Constant  Value=KDDM_DCDCDisPassSW_flg
  Constant15 : Constant  Value=KDDM_DCDCDisCFSSW_flg
  Constant16 : Constant  Value=TRUE
  Constant17 : Constant  Value=KDDM_DCDCDisPassTO_s
  Constant19 : Constant  Value=ENUM_POWERSTA_OFF
  Constant20 : Constant  Value=KDDM_DCDCDisDFSSW_flg
  Constant21 : Constant  Value=FALSE
  Constant22 : Constant  Value=ENUM_PWRSTASW_OFF
  Constant23 : Constant  Value=TRUE
  Constant24 : Constant  Value=TRUE
  Constant25 : Constant  Value=FALSE
  Constant27 : Constant  Value=FALSE
  Constant38 : Constant  Commented=on  Value=KDDM_DCDCDisDetTO_s
  Constant40 : Constant  Commented=on  Value=KDDM_DCDCDisDTC_cnt
  Constant43 : Constant  Value=KDDM_DCDCDisPassTO_s
  Constant44 : Constant  Value=KDDM_DCDCDisDetSW_flg
  DTC_Couter : hcu_lib/Basic_Blocks/DTC_Couter
  DTC_Info : hcu_lib/Basic_Blocks/DTC_Info
  Data Type Conversion1 : DataTypeConversion  OutDataTypeStr=uint8
  Equal1 : RelationalOperator  Operator===  OutDataTypeStr=boolean  RndMeth=Simplest
  Equal2 : RelationalOperator  Operator=~=  OutDataTypeStr=boolean  RndMeth=Simplest
  Equal4 : RelationalOperator  Operator=~=  OutDataTypeStr=boolean  RndMeth=Simplest
  Equal6 : RelationalOperator  OutDataTypeStr=boolean  RndMeth=Simplest
  Equal7 : RelationalOperator  Operator===  OutDataTypeStr=boolean  RndMeth=Simplest
  From48 : From  Commented=on  GotoTag=task_time_s
  Goto24 : Goto  Commented=on  GotoTag=VDDM_EDriveSysErrVCUErr_flg
  Logical Operator{12,15,18..19} (4 alike) : Logic  AllPortsSameDT=off  OutDataTypeStr=boolean
  Logical Operator3 : Logic  Operator=OR  AllPortsSameDT=off  OutDataTypeStr=boolean
  Logical Operator6 : Logic  Operator=NOT  AllPortsSameDT=off  OutDataTypeStr=boolean
  Logical Operator8 : Logic  Operator=OR  AllPortsSameDT=off  OutDataTypeStr=boolean
  Relay : Relay  OnSwitchValue=ONE_INT  OffSwitchValue=ZERO_INT
  SR_Latch1 : Subsystem  mask(SR_Latch){}
      mask help: SR latch function.
  SR_Latch3 : hcu_lib/Basic_Blocks/SR_Latch
  SR_Latch4 : hcu_lib/Basic_Blocks/SR_Latch
  Switch{,1,4..5} (4 alike) : Switch  Criteria=u2 ~= 0
  Test Detection Criteria : hcu_lib/Basic_Blocks/Test Detection Criteria  Commented=on
  Timer1 : hcu_lib/Basic_Blocks/Timer
  VDDM_DCDCDisDTC_raw32 : Outport
  wires:
  VPMM_PowerSta_enum/1 -> [VPMM_PowerSta_enum]
  VPMM_PwrStaSW_enum/1 -> [VPMM_PwrStaSW_enum]
  task_time_s/1 -> [task_time_s]
  Switch5/1 -> [VDDM_DCDCDisDet_flg]  "VDDM_DCDCDisDet_flg"
  Logical Operator6/1 -> Timer1/1
  Logical Operator8/1 -> Switch4/2
  [VDDM_DCDCDisCFSRls_flg] -> Logical Operator3/2
  SR_Latch3/1 -> Logical Operator12/2
  Switch/1 -> Goto24/1
  From48/1 -> Test Detection Criteria/2
  Constant24/1 -> Switch4/1
  Logical Operator18/1 -> [VDDM_DCDCDisCFS_flg]
  Constant15/1 -> Logical Operator18/2
  Constant21/1 -> Switch/3
  [VDDM_DCDCDisDet_flg] -> Logical Operator19/1
  Data Type Conversion1/1 -> [VDDM_DCDCDisDTC_cnt]  "VDDM_DCDCDisDTC_cnt"
  Constant19/1 -> Equal7/2
  [VDDM_DCDCDisChk_flg] -> Switch5/1
  Logical Operator3/1 -> Logical Operator15/1
  [VDDM_DCDCDisCFS_flg] -> Switch/2
  Constant16/1 -> Switch/1
  Switch4/1 -> [VDDM_DCDCDisCFSRls_flg]
  Logical Operator19/1 -> DTC_Couter/1
  Constant25/1 -> Switch4/3
  Constant27/1 -> Switch5/3
  DTC_Couter/1 -> SR_Latch4/1
  [VDDM_DCDCDisPass_flg] -> Logical Operator3/1
  Logical Operator15/1 -> DTC_Couter/2
  Constant17/1 -> Equal6/2
  Equal6/1 -> SR_Latch1/1(set)
  Constant43/1 -> Timer1/4
  Logical Operator12/1 -> [VDDM_DCDCDisDFS_flg]
  [VPMM_PwrStaSW_enum] -> Equal4/1
  Constant11/1 -> Logical Operator15/2
  SR_Latch4/1 -> Logical Operator18/1
  DTC_Couter/2 -> Data Type Conversion1/1
  [VDDM_DCDCDisCFSRls_flg] -> SR_Latch4/2
  [VDDM_DCDCDisChk_flg] -> Switch1/1
  Constant23/1 -> Switch1/3
  [VDDM_DCDCDisDTC_cnt] -> Relay/1
  Constant44/1 -> Logical Operator19/2
  SR_Latch1/1(latched) -> [VDDM_DCDCDisPass_flg]
  [VPMM_PowerSta_enum] -> Equal7/1
  Equal4/1 -> Switch5/2
  Equal2/1 -> Switch1/2
  Constant20/1 -> Logical Operator12/1
  Switch1/1 -> Logical Operator6/1, SR_Latch1/2(reset), Timer1/2
  Constant22/1 -> Equal4/2
  Relay/1 -> SR_Latch3/1
  [task_time_s] -> Timer1/3
  Constant10/1 -> DTC_Couter/3
  Timer1/1 -> Equal6/1
  [DTC_clear_request] -> Logical Operator8/2
  Constant40/1 -> Test Detection Criteria/3
  [VPMM_PwrStaSW_enum] -> Equal2/1
  Constant1/1 -> Equal2/2
  Equal7/1 -> Logical Operator8/1
  VPMM_PowerDownFault_enum/1 -> Equal1/1
  Constant/1 -> Equal1/2
  DTC_clear_request/1 -> [DTC_clear_request]
  Equal1/1 -> [VDDM_DCDCDisChk_flg]
  DTC_Info/1 -> VDDM_DCDCDisDTC_raw32/1  "VDDM_DCDCDisDTC_raw32"
  [VDDM_DCDCDisPass_flg] -> DTC_Info/2
  [VDDM_DCDCDisCFS_flg] -> DTC_Info/3
  [VDDM_DCDCDisCFS_flg] -> SR_Latch3/2
  [VDDM_DCDCDisDet_flg] -> DTC_Info/1
  Constant38/1 -> Test Detection Criteria/4
  [DTC_clear_request] -> DTC_Info/4

== system ddm/DDM/DDM/PMM/power up and power down/DCDC enable fail ==
  note: Release Condition After Failure Decision
  note: Test Detection Criteria
  note: Test Pass Criteria
  note: Release Condition During Failure Detection
  note: Diagnostics and Fault Handling
  note: Fail Safe Operation During Failure Detection
  note: Fail Safe Operation After Failure Decision
  task_time_s : Inport
  VPMM_PowerSta_enum : Inport  Port=2
  VPMM_PwrStaSW_enum : Inport  Port=3
  VINP_DCDCEnabled_flg : Inport  Port=4
  VPMM_PowerUpFault_enum : Inport  Port=5
  DTC_clear_request : Inport  Port=6
  VPMM_PowerUpState_enum : Inport  Port=7
  Constant : Constant  Value=ENUM_PUFAULT_DCDCENABLEFAIL
  Constant1 : Constant  Value=ENUM_PUSTATE_COMPLETED
  Constant10 : Constant  Value=KDDM_DCDCEnaDTC_cnt
  Constant11 : Constant  Value=KDDM_DCDCEnaPassSW_flg
  Constant15 : Constant  Value=KDDM_DCDCEnaCFSSW_flg
  Constant16 : Constant  Value=TRUE
  Constant19 : Constant  Value=ENUM_POWERSTA_OFF
  Constant{2,21,25,27} (4 alike) : Constant  Value=FALSE
  Constant20 : Constant  Value=KDDM_DCDCEnaDFSSW_flg
  Constant23 : Constant  Value=TRUE
  Constant24 : Constant  Value=TRUE
  Constant26 : Constant  Value=ENUM_PWRSTASW_OFF
  Constant38 : Constant  Commented=on  Value=KDDM_DCDCEnaDetTO_s
  Constant40 : Constant  Commented=on  Value=KDDM_DCDCEnaDTC_cnt
  Constant43 : Constant  Value=KDDM_DCDCEnaPassTO_s
  Constant44 : Constant  Value=KDDM_DCDCEnaDetSW_flg
  Constant8 : Constant  Value=KDDM_DCDCEnaPassTO_s
  DTC_Couter : hcu_lib/Basic_Blocks/DTC_Couter
  DTC_Info : hcu_lib/Basic_Blocks/DTC_Info
  Data Type Conversion1 : DataTypeConversion  OutDataTypeStr=uint8
  Equal : RelationalOperator  Operator=~=  OutDataTypeStr=boolean  RndMeth=Simplest
  Equal1 : RelationalOperator  Operator===  OutDataTypeStr=boolean  RndMeth=Simplest
  Equal2 : RelationalOperator  Operator===  OutDataTypeStr=boolean  RndMeth=Simplest
  Equal5 : RelationalOperator  OutDataTypeStr=boolean  RndMeth=Simplest
  Equal6 : RelationalOperator  Operator===  OutDataTypeStr=boolean  RndMeth=Simplest
  From48 : From  Commented=on  GotoTag=task_time_s
  Goto24 : Goto  Commented=on  GotoTag=VDDM_EDriveSysErrVCUErr_flg
  Logical Operator{5,12,15,18..19} (5 alike) : Logic  AllPortsSameDT=off  OutDataTypeStr=boolean
  Logical Operator3 : Logic  Operator=OR  AllPortsSameDT=off  OutDataTypeStr=boolean
  Logical Operator4 : Logic  Operator=NOT  AllPortsSameDT=off  OutDataTypeStr=boolean
  Logical Operator6 : Logic  Operator=NOT  AllPortsSameDT=off  OutDataTypeStr=boolean
  Logical Operator8 : Logic  Operator=OR  AllPortsSameDT=off  OutDataTypeStr=boolean
  Relay : Relay  OnSwitchValue=ONE_INT  OffSwitchValue=ZERO_INT
  SR_Latch1 : Subsystem  mask(SR_Latch){}
      mask help: SR latch function.
  SR_Latch3 : hcu_lib/Basic_Blocks/SR_Latch
  SR_Latch4 : hcu_lib/Basic_Blocks/SR_Latch
  Switch{,2,4..5} (4 alike) : Switch  Criteria=u2 ~= 0
  Test Detection Criteria : hcu_lib/Basic_Blocks/Test Detection Criteria  Commented=on
  Timer1 : hcu_lib/Basic_Blocks/Timer
  VDDM_DCDCEnaDTC_raw32 : Outport
  wires:
  task_time_s/1 -> [task_time_s]
  VPMM_PwrStaSW_enum/1 -> [VPMM_PwrStaSW_enum]
  VPMM_PowerSta_enum/1 -> [VPMM_PowerSta_enum]
  Logical Operator18/1 -> [VDDM_DCDCEnaCFS_flg]
  Constant21/1 -> Switch/3
  Equal5/1 -> SR_Latch1/1(set)
  Switch4/1 -> [VDDM_DCDCEnaCFSRls_flg]
  Data Type Conversion1/1 -> [VDDM_DCDCEnaDTC_cnt]  "VDDM_DCDCEnaDTC_cnt"
  Constant8/1 -> Equal5/2
  Constant20/1 -> Logical Operator12/1
  Logical Operator12/1 -> [VDDM_DCDCEnaDFS_flg]
  Constant15/1 -> Logical Operator18/2
  [task_time_s] -> Timer1/3
  DTC_Couter/1 -> SR_Latch4/1
  [VDDM_DCDCEnaCFSRls_flg] -> Logical Operator3/2
  Logical Operator19/1 -> DTC_Couter/1
  [VPMM_PowerSta_enum] -> Equal6/1
  [VDDM_DCDCEnaPass_flg] -> Logical Operator3/1
  Constant23/1 -> Switch2/3
  Constant16/1 -> Switch/1
  Constant26/1 -> Equal/2
  SR_Latch3/1 -> Logical Operator12/2
  From48/1 -> Test Detection Criteria/2
  Switch/1 -> Goto24/1
  Switch5/1 -> [VDDM_DCDCEnaDet_flg]  "VDDM_DCDCEnaDet_flg"
  [VDDM_DCDCEnaDet_flg] -> Logical Operator19/1
  Logical Operator3/1 -> Logical Operator15/1
  Constant24/1 -> Switch4/1
  SR_Latch4/1 -> Logical Operator18/1
  Logical Operator15/1 -> DTC_Couter/2
  Constant10/1 -> DTC_Couter/3
  Constant40/1 -> Test Detection Criteria/3
  Constant25/1 -> Switch4/3
  [VPMM_PwrStaSW_enum] -> Equal/1
  Relay/1 -> SR_Latch3/1
  [VDDM_DCDCEnaCFS_flg] -> Switch/2
  [DTC_clear_request] -> Logical Operator8/2
  Constant11/1 -> Logical Operator15/2
  [VDDM_DCDCEnaDTC_cnt] -> Relay/1
  Equal2/1 -> Switch2/2
  Equal/1 -> Switch5/2
  Logical Operator8/1 -> Switch4/2
  Logical Operator6/1 -> Timer1/1
  SR_Latch1/1(latched) -> [VDDM_DCDCEnaPass_flg]
  Equal6/1 -> Logical Operator8/1
  Constant27/1 -> Switch5/3
  Constant43/1 -> Timer1/4
  DTC_Couter/2 -> Data Type Conversion1/1
  Constant44/1 -> Logical Operator19/2
  Constant19/1 -> Equal6/2
  [VDDM_DCDCEnaChk_flg] -> Switch5/1
  Timer1/1 -> Equal5/1
  Switch2/1 -> SR_Latch1/2(reset), Timer1/2, Logical Operator6/1
  [VDDM_DCDCEnaCFSRls_flg] -> SR_Latch4/2
  DTC_clear_request/1 -> [DTC_clear_request]
  Constant/1 -> Equal1/2
  Equal1/1 -> Logical Operator5/2
  Logical Operator4/1 -> Logical Operator5/1
  VINP_DCDCEnabled_flg/1 -> Logical Operator4/1
  VPMM_PowerUpFault_enum/1 -> Equal1/1
  Logical Operator5/1 -> [VDDM_DCDCEnaChk_flg]
  DTC_Info/1 -> VDDM_DCDCEnaDTC_raw32/1  "VDDM_DCDCEnaDTC_raw32"
  [VDDM_DCDCEnaPass_flg] -> DTC_Info/2
  [VDDM_DCDCEnaCFS_flg] -> DTC_Info/3
  [VDDM_DCDCEnaCFS_flg] -> SR_Latch3/2
  [VDDM_DCDCEnaDet_flg] -> DTC_Info/1
  Constant38/1 -> Test Detection Criteria/4
  [DTC_clear_request] -> DTC_Info/4
  VPMM_PowerUpState_enum/1 -> [VPMM_PowerUpState_enum]
  Constant2/1 -> Switch2/1
  Constant1/1 -> Equal2/2
  [VPMM_PowerUpState_enum] -> Equal2/1

== system ddm/DDM/DDM/PMM/power up and power down/DCDC ready for precharge fail ==
  note: Release Condition During Failure Detection
  note: Test Detection Criteria
  note: Release Condition After Failure Decision
  note: Test Pass Criteria
  note: Fail Safe Operation After Failure Decision
  note: Fail Safe Operation During Failure Detection
  note: Diagnostics and Fault Handling
  task_time_s : Inport
  VPMM_PowerSta_enum : Inport  Port=2
  VPMM_PwrStaSW_enum : Inport  Port=3
  VINP_DCDCReady4Pre_flg : Inport  Port=4
  VPMM_PowerUpFault_enum : Inport  Port=5
  VINP_ReqClrDTC_flg : Inport  Port=6
  VPMM_PowerUpState_enum : Inport  Port=7
  Constant : Constant  Value=ENUM_PUFAULT_PRECHRGCHKFAIL
  Constant1 : Constant  Value=ENUM_PUSTATE_COMPLETED
  Constant10 : Constant  Value=KDDM_DCDC4PreDTC_cnt
  Constant11 : Constant  Value=KDDM_DCDC4PrePassSW_flg
  Constant15 : Constant  Value=KDDM_DCDC4PreCFSSW_flg
  Constant16 : Constant  Value=TRUE
  Constant19 : Constant  Value=ENUM_POWERSTA_OFF
  Constant{2,21,25,27} (4 alike) : Constant  Value=FALSE
  Constant20 : Constant  Value=KDDM_DCDC4PreDFSSW_flg
  Constant23 : Constant  Value=TRUE
  Constant24 : Constant  Value=TRUE
  Constant26 : Constant  Value=ENUM_PWRSTASW_OFF
  Constant38 : Constant  Commented=on  Value=KDDM_DCDC4PreDetTO_s
  Constant40 : Constant  Commented=on  Value=KDDM_DCDC4PreDTC_cnt
  Constant43 : Constant  Value=KDDM_DCDC4PrePassTO_s
  Constant44 : Constant  Value=KDDM_DCDC4PreDetSW_flg
  Constant8 : Constant  Value=KDDM_DCDC4PrePassTO_s
  DTC_Couter : hcu_lib/Basic_Blocks/DTC_Couter
  DTC_Info : hcu_lib/Basic_Blocks/DTC_Info
  Data Type Conversion1 : DataTypeConversion  OutDataTypeStr=uint8
  Equal : RelationalOperator  Operator=~=  OutDataTypeStr=boolean  RndMeth=Simplest
  Equal1 : RelationalOperator  Operator===  OutDataTypeStr=boolean  RndMeth=Simplest
  Equal2 : RelationalOperator  Operator===  OutDataTypeStr=boolean  RndMeth=Simplest
  Equal5 : RelationalOperator  OutDataTypeStr=boolean  RndMeth=Simplest
  Equal6 : RelationalOperator  Operator===  OutDataTypeStr=boolean  RndMeth=Simplest
  From48 : From  Commented=on  GotoTag=task_time_s
  Goto24 : Goto  Commented=on  GotoTag=VDDM_EDriveSysErrVCUErr_flg
  Logical Operator{5,12,15,18..19} (5 alike) : Logic  AllPortsSameDT=off  OutDataTypeStr=boolean
  Logical Operator3 : Logic  Operator=OR  AllPortsSameDT=off  OutDataTypeStr=boolean
  Logical Operator4 : Logic  Operator=NOT  AllPortsSameDT=off  OutDataTypeStr=boolean
  Logical Operator6 : Logic  Operator=NOT  AllPortsSameDT=off  OutDataTypeStr=boolean
  Logical Operator8 : Logic  Operator=OR  AllPortsSameDT=off  OutDataTypeStr=boolean
  Relay : Relay  OnSwitchValue=ONE_INT  OffSwitchValue=ZERO_INT
  SR_Latch1 : Subsystem  mask(SR_Latch){}
      mask help: SR latch function.
  SR_Latch3 : hcu_lib/Basic_Blocks/SR_Latch
  SR_Latch4 : hcu_lib/Basic_Blocks/SR_Latch
  Switch{,2,4..5} (4 alike) : Switch  Criteria=u2 ~= 0
  Test Detection Criteria : hcu_lib/Basic_Blocks/Test Detection Criteria  Commented=on
  Timer1 : hcu_lib/Basic_Blocks/Timer
  VDDM_DCDC4PreDTC_raw32 : Outport
  wires:
  VPMM_PowerSta_enum/1 -> [VPMM_PowerSta_enum]
  VPMM_PwrStaSW_enum/1 -> [VPMM_PwrStaSW_enum]
  task_time_s/1 -> [task_time_s]
  [VDDM_DCDC4PreCFSRls_flg] -> SR_Latch4/2
  Switch2/1 -> SR_Latch1/2(reset), Timer1/2, Logical Operator6/1
  [VDDM_DCDC4PreChk_flg] -> Switch5/1
  Equal6/1 -> Logical Operator8/1
  Timer1/1 -> Equal5/1
  SR_Latch1/1(latched) -> [VDDM_DCDC4PrePass_flg]
  Constant19/1 -> Equal6/2
  Logical Operator6/1 -> Timer1/1
  Constant44/1 -> Logical Operator19/2
  DTC_Couter/2 -> Data Type Conversion1/1
  Constant27/1 -> Switch5/3
  Logical Operator8/1 -> Switch4/2
  [VDDM_DCDC4PreDTC_cnt] -> Relay/1
  Constant11/1 -> Logical Operator15/2
  Relay/1 -> SR_Latch3/1
  Equal/1 -> Switch5/2
  [DTC_clear_request] -> Logical Operator8/2
  [VDDM_DCDC4PreCFS_flg] -> Switch/2
  [VDDM_DCDC4PreDet_flg] -> Logical Operator19/1
  Switch5/1 -> [VDDM_DCDC4PreDet_flg]  "VDDM_DCDC4PreDet_flg"
  Logical Operator3/1 -> Logical Operator15/1
  [VPMM_PwrStaSW_enum] -> Equal/1
  Constant40/1 -> Test Detection Criteria/3
  Constant43/1 -> Timer1/4
  SR_Latch4/1 -> Logical Operator18/1
  Constant25/1 -> Switch4/3
  Logical Operator15/1 -> DTC_Couter/2
  Constant24/1 -> Switch4/1
  Constant16/1 -> Switch/1
  Constant23/1 -> Switch2/3
  Constant26/1 -> Equal/2
  Switch/1 -> Goto24/1
  SR_Latch3/1 -> Logical Operator12/2
  Constant10/1 -> DTC_Couter/3
  [VDDM_DCDC4PreCFSRls_flg] -> Logical Operator3/2
  [VPMM_PowerSta_enum] -> Equal6/1
  [VDDM_DCDC4PrePass_flg] -> Logical Operator3/1
  From48/1 -> Test Detection Criteria/2
  Logical Operator19/1 -> DTC_Couter/1
  DTC_Couter/1 -> SR_Latch4/1
  Equal2/1 -> Switch2/2
  Constant20/1 -> Logical Operator12/1
  Logical Operator12/1 -> [VDDM_DCDC4PreDFS_flg]
  Constant15/1 -> Logical Operator18/2
  [task_time_s] -> Timer1/3
  Constant8/1 -> Equal5/2
  Equal5/1 -> SR_Latch1/1(set)
  Logical Operator18/1 -> [VDDM_DCDC4PreCFS_flg]
  Constant21/1 -> Switch/3
  Switch4/1 -> [VDDM_DCDC4PreCFSRls_flg]
  Data Type Conversion1/1 -> [VDDM_DCDC4PreDTC_cnt]  "VDDM_DCDC4PreDTC_cnt"
  VINP_ReqClrDTC_flg/1 -> [DTC_clear_request]
  Equal1/1 -> Logical Operator5/2
  Constant/1 -> Equal1/2
  VPMM_PowerUpFault_enum/1 -> Equal1/1
  Logical Operator5/1 -> [VDDM_DCDC4PreChk_flg]
  VINP_DCDCReady4Pre_flg/1 -> Logical Operator4/1
  Logical Operator4/1 -> Logical Operator5/1
  DTC_Info/1 -> VDDM_DCDC4PreDTC_raw32/1  "VDDM_DCDC4PreDTC_raw32"
  [VDDM_DCDC4PrePass_flg] -> DTC_Info/2
  [VDDM_DCDC4PreCFS_flg] -> DTC_Info/3
  [VDDM_DCDC4PreCFS_flg] -> SR_Latch3/2
  [VDDM_DCDC4PreDet_flg] -> DTC_Info/1
  Constant38/1 -> Test Detection Criteria/4
  [DTC_clear_request] -> DTC_Info/4
  VPMM_PowerUpState_enum/1 -> [VPMM_PowerUpState_enum]
  Constant2/1 -> Switch2/1
  Constant1/1 -> Equal2/2
  [VPMM_PowerUpState_enum] -> Equal2/1
